simulink model "Simulation_Sound"  (R2024b)
settings: Solver=VariableStepAuto  StartTime=0.0  StopTime=10.0  RelTol=1e-3
libraries: dspfdesign x1
settings Model: Creator=castl  LastModifiedBy=castl

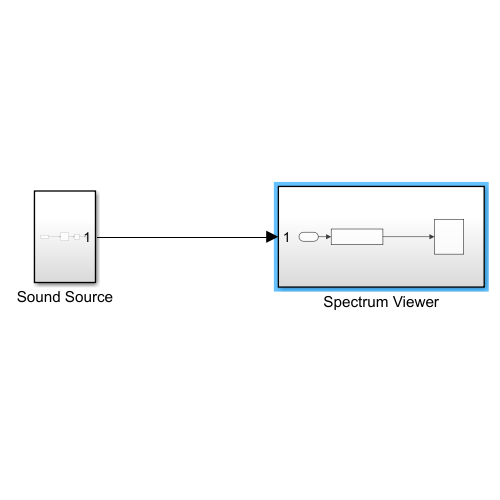
[thumbnail: Simulink's stored preview of the top-level diagram]
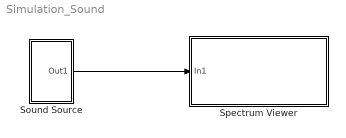
== system Simulation_Sound ==
  Sound Source : Subsystem
  Spectrum Viewer : Subsystem
  wires:
  Sound Source/1(Out1) -> Spectrum Viewer/1(In1)

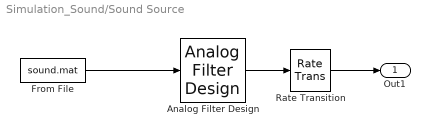
== system Simulation_Sound/Sound Source ==
  Analog Filter Design : dspfdesign/Analog Filter Design  method=Butterworth  filttype=Lowpass  N=8  Wlo=2*pi*4e3  Whi=80  Rp=2  Rs=40
  From File : FromFile  FileName=sound.mat  SampleTime=0
  Rate Transition : RateTransition
  Out1 : Outport
  wires:
  From File/1 -> Analog Filter Design/1
  Analog Filter Design/1 -> Rate Transition/1
  Rate Transition/1 -> Out1/1

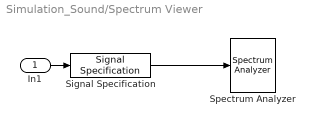
== system Simulation_Sound/Spectrum Viewer ==
  In1 : Inport
  Signal Specification : SignalSpecification  SampleTime=1/16e4
  Spectrum Analyzer : SpectrumAnalyzer  WindowPosition=[523.000000,651.000000,800.000000,500.000000,]  ScopeFrameLocation=window  Method=Welch  AxesScaling=Manual  FrequencyResolutionMethod=Window length  WindowInvariantSamplesPerUpdate=on  FrequencySpan=Span and center frequency  OverlapPercent=6.25  YLimits=[-40 25]  SelectedToolstripTab=spectrumAnalyzerToolstrip.estimationTab
  wires:
  Signal Specification/1 -> Spectrum Analyzer/1
  In1/1 -> Signal Specification/1
